simulink model "sampleModel2064"  (R2023a)
settings: Solver=VariableStepAuto  StartTime=0.0  StopTime=10.0  RelTol=1e-3
libraries: hdlsllib x5, simulink x1
settings Model: Creator=user1  LastModifiedBy=user1

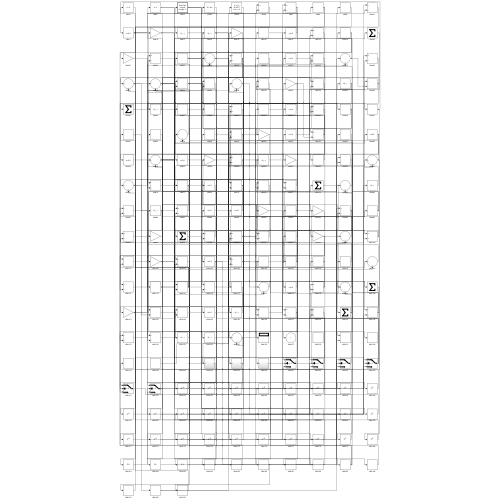
[thumbnail: Simulink's stored preview of the top-level diagram]
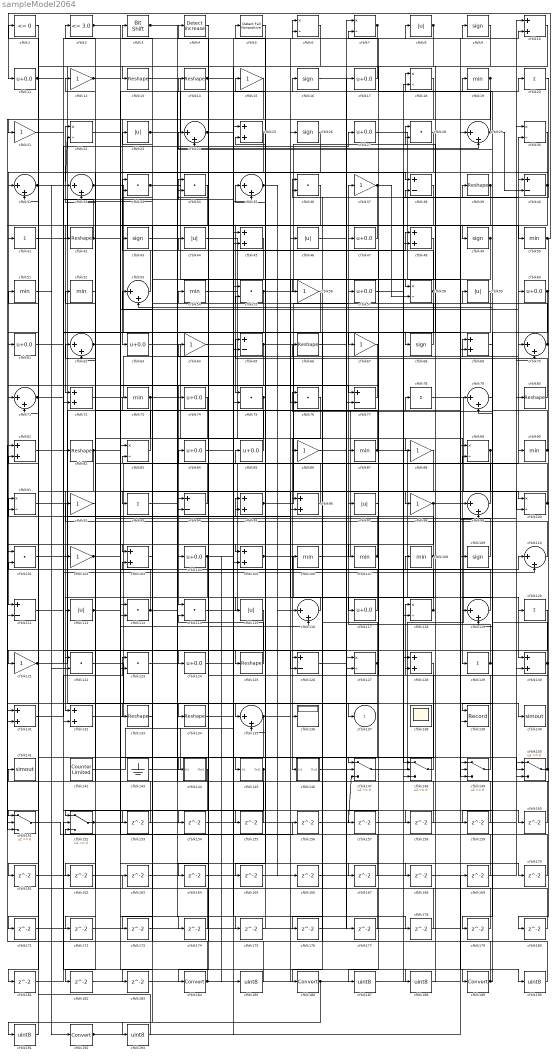
== system sampleModel2064 ==
  cfblk1 : hdlsllib/Logic and Bit Operations/Compare To Zero  relop=<=  OutDataTypeStr=boolean
  cfblk{10,25,45,48,69,72,81,95..96,103,105,128,130..132} (15 alike) : Sum
  cfblk{6..7,18,22,30,58,83,89,91,100,118,127} (12 alike) : Product  Inputs=*/  RndMeth=Zero  SaturateOnIntegerOverflow=on
  cfblk{28,33..34,36,55,75..76,101,113..114,122..123} (12 alike) : DotProduct  OutDataTypeStr=Inherit: Inherit via internal rule
  cfblk{12,15,21,37,56,64,67,86,88,92,98,102,121} (13 alike) : Gain
  cfblk{11,17,27,47,57,60..61,63,74,84..85,104,117,124} (14 alike) : Bias  Bias=0.0  SaturateOnIntegerOverflow=off
  cfblk{19,50..52,54,73,87,90,106..108} (11 alike) : MinMax
  cfblk{9,16,26,43,49,68,109} (7 alike) : Signum
  cfblk{24,29,31..32,35,53,62,70..71,79,99,110,116,119,135} (15 alike) : Sum  Inputs=|++
  cfblk{38,40,65,77,94,111,126} (7 alike) : Sum  Inputs=+-
  cfblk{8,23,44,46,59,97,112,115} (8 alike) : Abs  SaturateOnIntegerOverflow=off
  cfblk{20,41,78,93,120,129} (6 alike) : Sum  Inputs=+
  cfblk{13..14,39,42,66,80,82,125,133..134} (10 alike) : Reshape
  cfblk136 : Display
  cfblk138 : Scope
      settings: Floating=on
  cfblk139 : Record  FileSettingsInternal="{\"entries\":[{\"content\":{\"excelSettings\":{\"content\":{},\"type\":\"Streamout.ExcelSettings\"}},\"type\":\"Streamout.FileSettingStorage\",\"uuid\":\"\"}],\"packageUris\":[\"http:\\/\\/schema.mathworks.com\\/mf0\\/streamout_blocks\\/R2020a\"],\"version\":\"1.0\"}"  Layout=[1 1]  SignalsInternal="{\"entries\":[{\"content\":{},\"type\":\"RecordBlkView.InputSignals\",\"uuid\":\"\"}],\"packageUris\":[\"http:\\/\\/schema.mathworks.com\\/mf0\\/streamout_blocks\\/R2020a\"],\"version\":\"1.0\"}"  VisualizationBindings="{\"xyplotplugin\":{\"info\":[{\"series\":[{\"bindingParametersList\":[{\"parameter\":\"X-Axis\",\"signalID\":6435,\"signalName\":\"cfblk89\"},{\"parameter\":\"Y-Axis\",\"signalID\":6439,\"signalName\":\"cfblk33\"}],\"seriesID\":26884}],\"subplotID\":1}]}}"  CompatibilityTag=XY  st=-1
  cfblk140 : ToWorkspace  VariableName=simout  SaveFormat=Timeseries  SampleTime=-1
  cfblk141 : ToWorkspace  VariableName=simout  SaveFormat=Timeseries  SampleTime=-1
  cfblk142 : hdlsllib/Sources/Counter Limited  uplimit=7  tsamp=-1
  cfblk143 : Ground
  cfblk144 : Subsystem
      settings: LibrarySourceBlock=|
      | hdlsllib/Ports &
      | Subsystems/Subsystem
  cfblk145 : Subsystem
      settings: LibrarySourceBlock=|
      | hdlsllib/Ports &
      | Subsystems/Subsystem
  cfblk146 : Subsystem
      settings: LibrarySourceBlock=|
      | hdlsllib/Ports &
      | Subsystems/Subsystem
  cfblk{147..152} (6 alike) : Switch  SaturateOnIntegerOverflow=off  InputSameDT=off
  cfblk{153..183} (31 alike) : Delay  SampleTime=1
  cfblk{184,186,189,192} (4 alike) : DataTypeConversion  SaturateOnIntegerOverflow=off  RndMeth=Floor
  cfblk{185,187..188,190..191,193} (6 alike) : DataTypeConversion  OutDataTypeStr=uint8  SaturateOnIntegerOverflow=off  RndMeth=Floor
  cfblk2 : hdlsllib/Logic and Bit Operations/Compare To Constant  relop=<=  const=3.0  OutDataTypeStr=boolean
  cfblk3 : hdlsllib/Logic and Bit Operations/Bit Shift  mode=Shift Left Logical  N=0
  cfblk4 : simulink/Logic and Bit Operations/Detect Increase  vinit=0.0  OutDataTypeStr=boolean
      settings: LibrarySourceBlock=|
      | hdlsllib/Logic and Bit
      | Operations/Detect
      | Increase
  cfblk5 : hdlsllib/Logic and Bit Operations/Detect Fall Nonpositive  vinit=0  OutDataTypeStr=boolean
  cfblk137 : Outport  VectorParamsAs1DForOutWhenUnconnected=off
  wires:
  cfblk67/1 -> cfblk114/1
  cfblk100/1 -> cfblk84/1, cfblk93/1
  cfblk102/1 -> cfblk150/2, cfblk155/1
  cfblk8/1 -> cfblk134/1, cfblk21/1
  cfblk18/1 -> cfblk63/1
  cfblk132/1 -> cfblk85/1
  cfblk78/1 -> cfblk100/1
  cfblk25/1 -> cfblk102/1, cfblk122/1, cfblk154/1
  cfblk35/1 -> cfblk125/1, cfblk116/1
  cfblk63/1 -> cfblk146/1(In1)
  cfblk3/1 -> cfblk96/2, cfblk88/1, cfblk175/1
  cfblk125/1 -> cfblk54/1
  cfblk44/1 -> cfblk129/1
  cfblk24/1 -> cfblk35/2, cfblk127/2
  cfblk17/1 -> cfblk13/1
  cfblk130/1 -> cfblk118/1, cfblk24/1, cfblk76/1
  cfblk117/1 -> cfblk37/1
  cfblk106/1 -> cfblk78/1
  cfblk42/1 -> cfblk22/1, cfblk188/1
  cfblk103/1 -> cfblk133/1
  cfblk129/1 -> cfblk97/1, cfblk79/2
  cfblk31/1 -> cfblk22/2, cfblk122/2
  cfblk26/1 -> cfblk111/1
  cfblk94/1 -> cfblk2/1
  cfblk58/1 -> cfblk3/1, cfblk43/1, cfblk176/1
  cfblk38/1 -> cfblk72/1
  cfblk95/1 -> cfblk57/1, cfblk117/1
  cfblk40/1 -> cfblk31/1, cfblk42/1
  cfblk107/1 -> cfblk64/1, cfblk91/1
  cfblk20/1 -> cfblk39/1
  cfblk150/1 -> cfblk87/1, cfblk95/2, cfblk119/2
  cfblk50/1 -> cfblk11/1, cfblk180/1
  cfblk70/1 -> cfblk141/1, cfblk32/2
  cfblk66/1 -> cfblk127/1
  cfblk122/1 -> cfblk136/1
  cfblk55/1 -> cfblk28/1, cfblk72/2
  cfblk33/1 -> cfblk56/1, cfblk139/2, cfblk148/1
  cfblk135/1 -> cfblk8/1, cfblk161/1
  cfblk148/1 -> cfblk15/1
  cfblk62/1 -> cfblk140/1, cfblk60/1, cfblk75/2, cfblk158/1, cfblk174/1
  cfblk39/1 -> cfblk75/1, cfblk36/2
  cfblk53/1 -> cfblk33/1
  cfblk46/1 -> cfblk7/1
  cfblk32/1 -> cfblk67/1, cfblk38/1, cfblk77/2, cfblk126/1
  cfblk10/1 -> cfblk68/1
  cfblk73/1 -> cfblk96/1, cfblk162/1
  cfblk113/1 -> cfblk31/2, cfblk16/1, cfblk91/2, cfblk101/2
  cfblk54/1 -> cfblk77/1
  cfblk92/1 -> cfblk12/1
  cfblk109/1 -> cfblk62/1
  cfblk126/1 -> cfblk17/1
  cfblk142/1 -> cfblk45/1
  cfblk97/1 -> cfblk47/1
  cfblk91/1 -> cfblk29/1
  cfblk108/1 -> cfblk83/2, cfblk157/1
  cfblk114/1 -> cfblk30/2
  cfblk13/1 -> cfblk58/1
  cfblk147/1 -> cfblk80/1
  cfblk83/1 -> cfblk62/2
  cfblk77/1 -> cfblk71/1
  cfblk36/1 -> cfblk105/1
  cfblk12/1 -> cfblk74/1, cfblk48/2
  cfblk5/1 -> cfblk135/1
  cfblk72/1 -> cfblk69/1
  cfblk60/1 -> cfblk119/1, cfblk159/1
  cfblk133/1 -> cfblk23/1
  cfblk85/1 -> cfblk73/1
  cfblk152/1 -> cfblk99/2, cfblk147/3
  cfblk104/1 -> cfblk123/2, cfblk126/2, cfblk185/1
  cfblk30/1 -> cfblk145/1(In1)
  cfblk98/1 -> cfblk10/2, cfblk151/2, cfblk183/1
  cfblk1/1 -> cfblk121/1
  cfblk29/1 -> cfblk7/2, cfblk40/2
  cfblk121/1 -> cfblk70/1, cfblk34/2
  cfblk79/1 -> cfblk19/1
  cfblk51/1 -> cfblk192/1
  cfblk16/1 -> cfblk100/2
  cfblk119/1 -> cfblk44/1
  cfblk143/1 -> cfblk55/1
  cfblk99/1 -> cfblk55/2
  cfblk71/1 -> cfblk27/1, cfblk82/1
  cfblk68/1 -> cfblk25/2
  cfblk28/1 -> cfblk147/1
  cfblk14/1 -> cfblk49/1, cfblk50/1
  cfblk65/1 -> cfblk149/3, cfblk101/1
  cfblk37/1 -> cfblk111/2, cfblk58/2
  cfblk87/1 -> cfblk130/1, cfblk52/1
  cfblk11/1 -> cfblk6/1, cfblk9/1, cfblk69/2
  cfblk27/1 -> cfblk109/1
  cfblk88/1 -> cfblk132/1
  cfblk112/1 -> cfblk110/1, cfblk20/1
  cfblk128/1 -> cfblk186/1
  cfblk118/1 -> cfblk115/1, cfblk108/1
  cfblk47/1 -> cfblk41/1
  cfblk146/1(Out1) -> cfblk90/1
  cfblk75/1 -> cfblk144/1(In1), cfblk135/2
  cfblk19/1 -> cfblk113/2, cfblk151/3
  cfblk43/1 -> cfblk29/2
  cfblk115/1 -> cfblk151/1
  cfblk15/1 -> cfblk94/2
  cfblk49/1 -> cfblk104/1, cfblk76/2
  cfblk105/1 -> cfblk120/1, cfblk166/1
  cfblk110/1 -> cfblk92/1
  cfblk23/1 -> cfblk18/1, cfblk118/2, cfblk24/2
  cfblk34/1 -> cfblk103/1
  cfblk90/1 -> cfblk53/2, cfblk38/2
  cfblk81/1 -> cfblk189/1
  cfblk6/1 -> cfblk61/1
  cfblk80/1 -> cfblk65/1
  cfblk7/1 -> cfblk105/2, cfblk171/1
  cfblk9/1 -> cfblk107/1
  cfblk149/1 -> cfblk34/1
  cfblk82/1 -> cfblk14/1, cfblk181/1
  cfblk96/1 -> cfblk5/1
  cfblk59/1 -> cfblk132/2
  cfblk41/1 -> cfblk6/2
  cfblk76/1 -> cfblk86/1
  cfblk57/1 -> cfblk40/1
  cfblk124/1 -> cfblk48/1
  cfblk116/1 -> cfblk112/1
  cfblk145/1(Out1) -> cfblk152/1, cfblk95/1
  cfblk61/1 -> cfblk124/1
  cfblk134/1 -> cfblk89/2
  cfblk101/1 -> cfblk26/1
  cfblk4/1 -> cfblk184/1
  cfblk2/1 -> cfblk98/1, cfblk116/2
  cfblk84/1 -> cfblk66/1
  cfblk131/1 -> cfblk123/1
  cfblk127/1 -> cfblk36/1, cfblk131/2, cfblk164/1
  cfblk111/1 -> cfblk110/2
  cfblk89/1 -> cfblk139/1, cfblk137/1
  cfblk56/1 -> cfblk153/1
  cfblk153/1 -> cfblk32/1
  cfblk154/1 -> cfblk30/1
  cfblk155/1 -> cfblk94/1
  cfblk151/1 -> cfblk156/1
  cfblk156/1 -> cfblk130/2
  cfblk157/1 -> cfblk149/2
  cfblk158/1 -> cfblk25/1
  cfblk159/1 -> cfblk1/1
  cfblk21/1 -> cfblk160/1
  cfblk160/1 -> cfblk114/2
  cfblk161/1 -> cfblk18/2
  cfblk162/1 -> cfblk150/3
  cfblk163/1 -> cfblk70/2
  cfblk164/1 -> cfblk150/1
  cfblk120/1 -> cfblk165/1
  cfblk165/1 -> cfblk10/1
  cfblk166/1 -> cfblk148/2
  cfblk123/1 -> cfblk167/1
  cfblk167/1 -> cfblk83/1
  cfblk93/1 -> cfblk168/1
  cfblk169/1 -> cfblk28/2
  cfblk22/1 -> cfblk170/1
  cfblk170/1 -> cfblk113/1
  cfblk171/1 -> cfblk65/2
  cfblk74/1 -> cfblk172/1
  cfblk172/1 -> cfblk79/1
  cfblk45/1 -> cfblk173/1
  cfblk173/1 -> cfblk99/1
  cfblk174/1 -> cfblk152/3
  cfblk175/1 -> cfblk35/1
  cfblk176/1 -> cfblk147/2
  cfblk86/1 -> cfblk177/1
  cfblk177/1 -> cfblk71/2
  cfblk64/1 -> cfblk178/1
  cfblk178/1 -> cfblk33/2
  cfblk69/1 -> cfblk179/1
  cfblk179/1 -> cfblk53/1
  cfblk180/1 -> cfblk103/2
  cfblk181/1 -> cfblk152/2
  cfblk52/1 -> cfblk182/1
  cfblk182/1 -> cfblk149/1
  cfblk183/1 -> cfblk148/3
  cfblk184/1 -> cfblk131/1, cfblk46/1
  cfblk185/1 -> cfblk4/1
  cfblk186/1 -> cfblk169/1, cfblk191/1
  cfblk48/1 -> cfblk187/1
  cfblk187/1 -> cfblk128/1
  cfblk188/1 -> cfblk128/2
  cfblk189/1 -> cfblk163/1, cfblk106/1, cfblk59/1
  cfblk168/1 -> cfblk190/1
  cfblk190/1 -> cfblk81/1
  cfblk191/1 -> cfblk81/2
  cfblk192/1 -> cfblk45/2, cfblk89/1
  cfblk144/1(Out1) -> cfblk193/1
  cfblk193/1 -> cfblk51/1

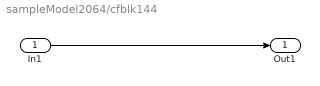
== system sampleModel2064/cfblk144 ==
  In1 : Inport
  Out1 : Outport
  wires:
  In1/1 -> Out1/1

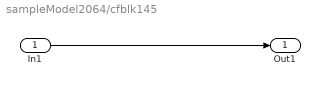
== system sampleModel2064/cfblk145 ==
  In1 : Inport
  Out1 : Outport
  wires:
  In1/1 -> Out1/1

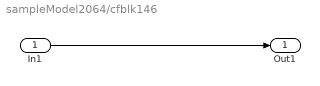
== system sampleModel2064/cfblk146 ==
  In1 : Inport
  Out1 : Outport
  wires:
  In1/1 -> Out1/1
